simulink model "problem_01_simul"  (R2018b)
settings: Solver=VariableStepAuto  StartTime=0.0  StopTime=10.0  RelTol=1e-3
libraries: cstblocks x1
settings Model: Creator=fabio  LastModifiedBy=fabio

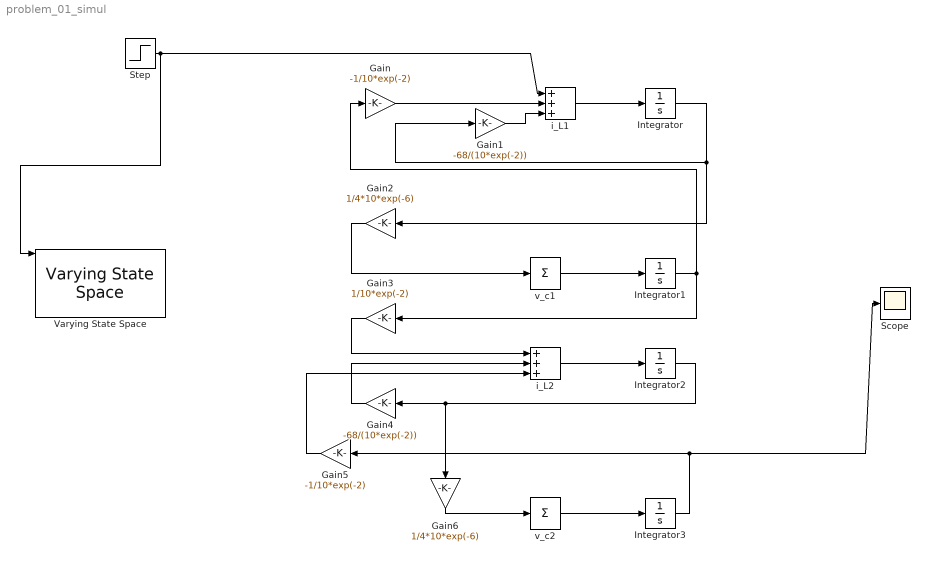
== system problem_01_simul ==
  Gain : Gain  Gain=-1/10*exp(-2)
  Gain1 : Gain  Gain=-68/(10*exp(-2))
  Gain2 : Gain  Gain=1/4*10*exp(-6)
  Gain3 : Gain  Gain=1/10*exp(-2)
  Gain4 : Gain  Gain=-68/(10*exp(-2))
  Gain5 : Gain  Gain=-1/10*exp(-2)
  Gain6 : Gain  Gain=1/4*10*exp(-6)
  Integrator{,1..3} (4 alike) : Integrator
  Scope : Scope
  Step : Step  Time=0  SampleTime=0
  Varying State Space : cstblocks/Linear Parameter Varying/Varying State Space  x0=0  xNames=''  OutputX=on  OutputDX=on
      settings: SourceProductName=Control System Toolbox
  i_L1 : Sum  Inputs=+++
  i_L2 : Sum  Inputs=+++
  v_c1 : Sum  Inputs=+
  v_c2 : Sum  Inputs=+
  wires:
  Step/1 -> Varying State Space/1, i_L1/1
  i_L1/1 -> Integrator/1
  i_L2/1 -> Integrator2/1
  v_c1/1 -> Integrator1/1
  v_c2/1 -> Integrator3/1
  Integrator1/1 -> Gain3/1, Gain/1
  Gain/1 -> i_L1/2
  Integrator/1 -> Gain2/1, Gain1/1
  Gain1/1 -> i_L1/3
  Gain2/1 -> v_c1/1
  Gain3/1 -> i_L2/1
  Integrator2/1 -> Gain6/1, Gain4/1
  Gain4/1 -> i_L2/2
  Integrator3/1 -> Scope/1, Gain5/1
  Gain5/1 -> i_L2/3
  Gain6/1 -> v_c2/1
